simulink model "task3_output_y_func"  (R2021b)
settings: Solver=FixedStepAuto  StartTime=0.0  StopTime=3  FixedStep=0.0001  RelTol=1e-3
settings Model: Creator=den  LastModifiedBy=den

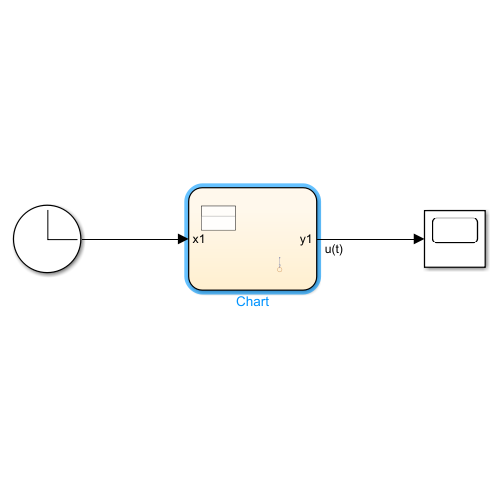
[thumbnail: Simulink's stored preview of the top-level diagram]
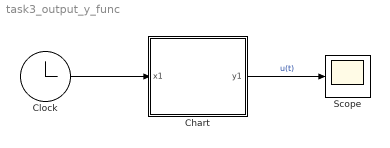
== system task3_output_y_func ==
  Chart : Stateflow chart  TreatAsAtomicUnit=on
  Clock : Clock
  Scope : Scope
  wires:
  Clock/1 -> Chart/1(x1)
  Chart/1(y1) -> Scope/1  "u(t)"

== matlab function task3_output_y_func/Chart ==
  data: x function_input; y function_output; x1 input; y1 output
function y = u(x)
    y = (-3 .* exp(-4 .* x)) .* cos(2 .* x) + (2 .* exp(-4  .* x)) .* sin(2 .* x);
end
